simulink model "Simulink_joaco"  (R2016a)
settings: Solver=VariableStepAuto  StartTime=0.0  StopTime=5  RelTol=1e-3
settings Model: Creator=joa-m  LastModifiedBy=Marcelo

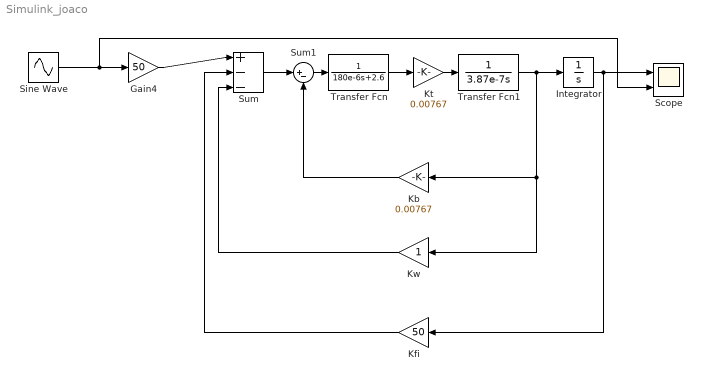
== system Simulink_joaco ==
  Gain4 : Gain  Gain=50
  Integrator : Integrator
  "Kb " : Gain  Gain=0.00767
  Kfi : Gain  Gain=50
  Kt : Gain  Gain=0.00767
  Kw : Gain
  Scope : Scope  NumInputPorts=2
  Sine Wave : Sin  Amplitude=2.5  Bias=2.50  Frequency=1.25  Phase=-1.5708  SampleTime=0
  Sum : Sum  Inputs=|+--
  Sum1 : Sum  Inputs=|+-
  Transfer Fcn : TransferFcn  Denominator=[180e-6 2.6]
  Transfer Fcn1 : TransferFcn  Denominator=[3.87e-7 0]
  wires:
  Sum/1 -> Sum1/1
  Integrator/1 -> Scope/1, Kfi/1
  Transfer Fcn1/1 -> "Kb "/1, Kw/1, Integrator/1
  "Kb "/1 -> Sum1/2
  Kw/1 -> Sum/3
  Kfi/1 -> Sum/2
  Gain4/1 -> Sum/1
  Sine Wave/1 -> Scope/2, Gain4/1
  Transfer Fcn/1 -> Kt/1
  Sum1/1 -> Transfer Fcn/1
  Kt/1 -> Transfer Fcn1/1
